simulink model "constant_complex_test"  (Simulink 8.4)
settings: Solver=ode45  StartTime=0.0  StopTime=10.0  RelTol=1e-3
settings Model: Creator=arnaud  LastModifiedBy=arnaud
settings DataIOCC: SaveFormat=Structure

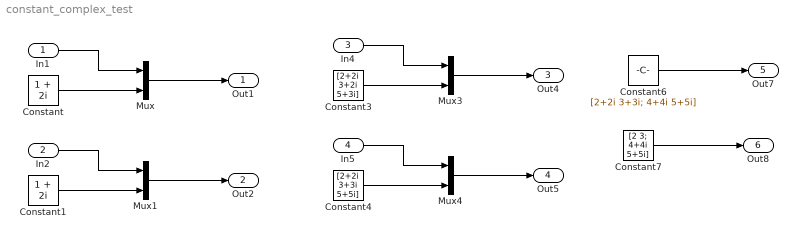
== system constant_complex_test ==
  In1 : Inport  OutDataTypeStr=double
  In2 : Inport  Port=2  OutDataTypeStr=int8
  In4 : Inport  Port=3  OutDataTypeStr=double
  In5 : Inport  Port=4  OutDataTypeStr=int8
  Constant : Constant  Value=1 + 2i  OutDataTypeStr=double
  Constant1 : Constant  Value=1 + 2i  OutDataTypeStr=int8
  Constant3 : Constant  Value=[2+2i 3+2i 5+3i]  OutDataTypeStr=double
  Constant4 : Constant  Value=[2+2i 3+3i 5+5i]  OutDataTypeStr=int8
  Constant6 : Constant  Value=[2+2i 3+3i; 4+4i 5+5i]  OutDataTypeStr=double
  Constant7 : Constant  Value=[2 3; 4+4i 5+5i]  OutDataTypeStr=int8
  Mux{,1,3..4} (4 alike) : Mux  Inputs=2
  Out1 : Outport
  Out2 : Outport  Port=2
  Out4 : Outport  Port=3
  Out5 : Outport  Port=4
  Out7 : Outport  Port=5
  Out8 : Outport  Port=6
  wires:
  In1/1 -> Mux/1
  Constant/1 -> Mux/2
  Mux/1 -> Out1/1
  In2/1 -> Mux1/1
  Constant1/1 -> Mux1/2
  Mux1/1 -> Out2/1
  In4/1 -> Mux3/1
  Constant3/1 -> Mux3/2
  Mux3/1 -> Out4/1
  In5/1 -> Mux4/1
  Constant4/1 -> Mux4/2
  Mux4/1 -> Out5/1
  Constant6/1 -> Out7/1
  Constant7/1 -> Out8/1
